simulink model "Task_2b"  (R2021b)
settings: Solver=VariableStepAuto  StartTime=0.0  StopTime=10.0  RelTol=1e-3
model workspace (MAT data in the model file):
  J = 0.01
  K = 0.01
  Kd = 1
  Ki = 60
  Kp = 50
  Kt = 1
  L = 0.5
  R = 1
  Ts = 0.01
  b = 0.1
  u = 25
settings Model: Creator=mluser  LastModifiedBy=mluser

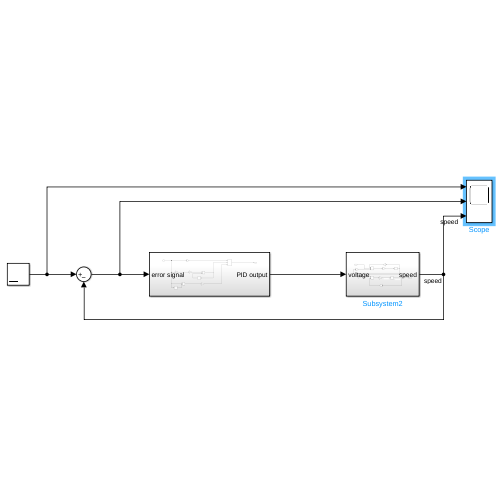
[thumbnail: Simulink's stored preview of the top-level diagram]
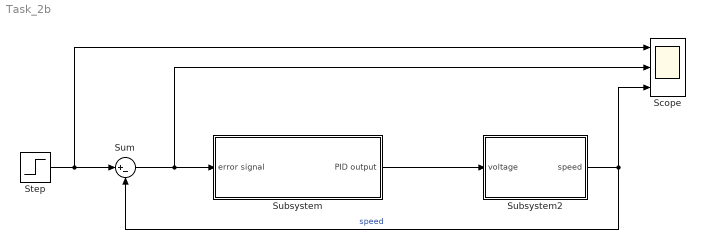
== system Task_2b ==
  Scope : Scope  NumInputPorts=3
  Step : Step  Time=0  After=u  SampleTime=0.01
  Subsystem : Subsystem
  Subsystem2 : Subsystem
  Sum : Sum  Inputs=|+-
  wires:
  Step/1 -> Sum/1, Scope/1
  Subsystem/1(PID output) -> Subsystem2/1(voltage)
  Subsystem2/1(speed) -> Scope/3, Sum/2  "speed"
  Sum/1 -> Subsystem/1(error signal), Scope/2

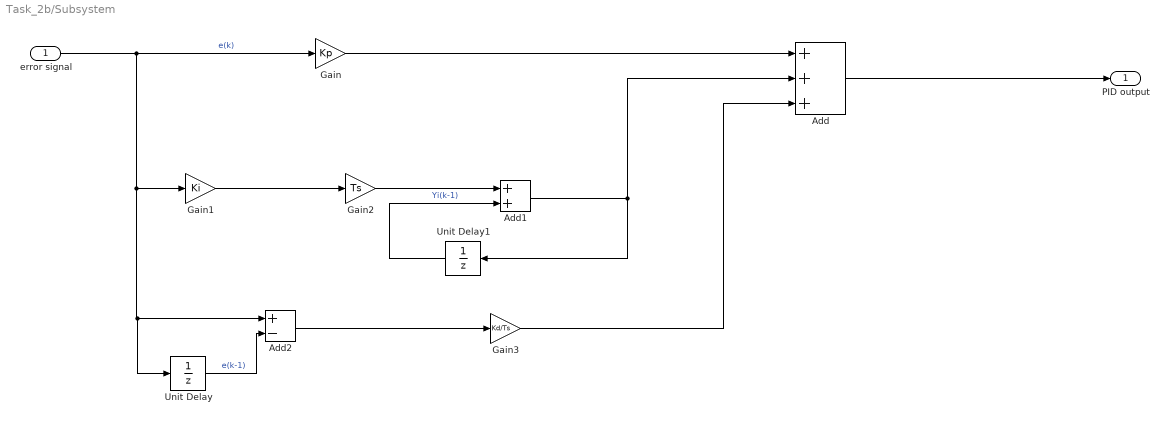
== system Task_2b/Subsystem ==
  error signal : Inport
  Add : Sum  Inputs=+++
  Add1 : Sum
  Add2 : Sum  Inputs=+-
  Gain : Gain  Gain=Kp
  Gain1 : Gain  Gain=Ki
  Gain2 : Gain  Gain=Ts
  Gain3 : Gain  Gain=Kd/Ts
  Unit Delay : UnitDelay  SampleTime=-1  HasFrameUpgradeWarning=on
  Unit Delay1 : UnitDelay  SampleTime=-1  HasFrameUpgradeWarning=on
  PID output : Outport
  wires:
  Unit Delay1/1 -> Add1/2  "Yi(k-1)"
  Gain3/1 -> Add/3
  Gain1/1 -> Gain2/1
  Unit Delay/1 -> Add2/2  "e(k-1)"
  Gain/1 -> Add/1
  error signal/1 -> Unit Delay/1, Add2/1, Gain1/1, Gain/1  "e(k)"
  Add/1 -> PID output/1
  Add2/1 -> Gain3/1
  Add1/1 -> Add/2, Unit Delay1/1
  Gain2/1 -> Add1/1

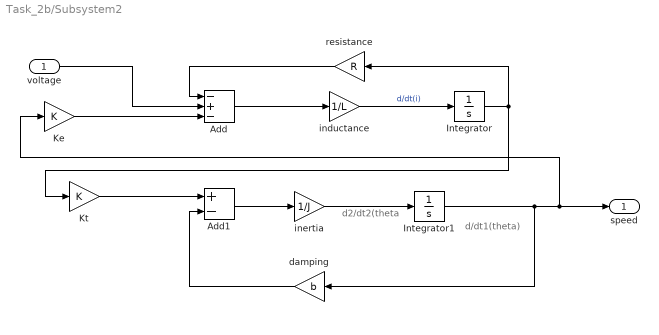
== system Task_2b/Subsystem2 ==
  note: d/dt1(theta)
  note: d2/dt2(theta
  voltage : Inport
  Add : Sum  Inputs=-+-
  Add1 : Sum  Inputs=+-
  Integrator : Integrator
  Integrator1 : Integrator
  Ke : Gain  Gain=K
  Kt : Gain  Gain=K
  damping : Gain  Gain=b
  "inductance " : Gain  Gain=1/L
  inertia : Gain  Gain=1/J
  resistance : Gain  Gain=R
  speed : Outport
  wires:
  Add1/1 -> inertia/1
  voltage/1 -> Add/2
  Integrator1/1 -> speed/1, Ke/1, damping/1
  "inductance "/1 -> Integrator/1  "d/dt(i)"
  damping/1 -> Add1/2
  inertia/1 -> Integrator1/1
  Integrator/1 -> resistance/1, Kt/1
  Kt/1 -> Add1/1
  Add/1 -> "inductance "/1
  Ke/1 -> Add/3
  resistance/1 -> Add/1
